simulink model "longitudinal_new"  (R2019a)
settings: Solver=VariableStepAuto  StartTime=0.0  StopTime=2000  RelTol=1e-3
values from neighbouring files (symbols this model uses):
  A = [-0.0804 0.1665 0 -9.8100 0 ... (first row only)    [longitudinaloia.m]    (also in oia.m = [-0.1245 0.0350 0.0414 -0.9962 0; -15.2138 -2.0587 0.0032 0.; state_space2tf.m = [-0.0558 -0.9968 0.0802 0.0415;0.5980 -0.1150 -0.0318 0;-3.0)
  B = [0 32.1224 ... (first row only)    [longitudinaloia.m]    (also in oia.m = [-0.0049 0.0237 ;-4.0379 0.9613; 0   0  ; -0.0568 -1.2168; 0; state_space2tf.m = [0.0073 0; -0.4750    0.0077;  0.1530    0.1430;0         0])
  C = [1          0          0          0 0;  0          1       0          0 0 ; 0       0          1          0 0; 0  0    0        1 0; 0 0 0 0 1]    [longitudinaloia.m]    (also in oia.m; state_space2tf.m = [0     1     0     0;  0     0     0     1])
  D = [0 0 ;0 0 ; 0 0 ;0   0;0 0]    [longitudinaloia.m]    (also in oia.m; state_space2tf.m = [0 0; 0 0])
libraries: simulink x3
settings Model: Creator=admin  LastModifiedBy=admin

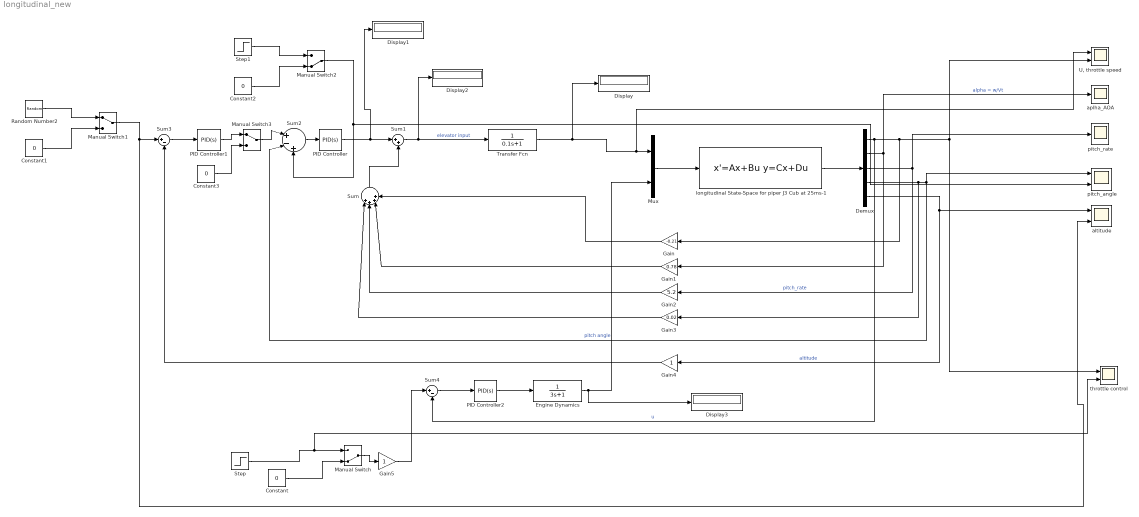
== system longitudinal_new ==
  " throttle control" : Scope  NumInputPorts=2
  Constant{,1..3} (4 alike) : Constant  Value=0
  Demux : Demux  Outputs=5
  Display{,1..3} (4 alike) : Display
  Engine Dynamics : TransferFcn  Denominator=[3 1]
  Gain : Gain  Gain=-0.21
  Gain1 : Gain  Gain=0.78
  Gain2 : Gain  Gain=5.2
  Gain3 : Gain  Gain=0.02
  Gain4 : Gain
  Gain5 : Gain
  Manual Switch : ManualSwitch  CurrentSetting=0
  Manual Switch1 : ManualSwitch
  Manual Switch2 : ManualSwitch  CurrentSetting=0
  Manual Switch3 : ManualSwitch
  Mux : Mux  Inputs=2
  PID Controller : simulink/Continuous/PID Controller  Controller=PID  Form=Parallel  TimeDomain=Continuous-time  SampleTime=-1  IntegratorMethod=Forward Euler  FilterMethod=Forward Euler  ControllerParametersSource=internal  P=0.45  I=0.4  D=0  UseFilter=on  N=100  TunerSelectOption=Transfer Function Based (PID Tuner App)  InitialConditionSource=internal  InitialConditionForIntegrator=0  InitialConditionForFilter=0  DifferentiatorICPrevScaledInput=0  ExternalReset=none  TrackingMode=off  Kt=1  LimitOutput=off  UpperSaturationLimit=inf  LowerSaturationLimit=-inf  LinearizeAsGain=on  AntiWindupMode=none  Kb=1  POutMin=[]  POutMax=[]  IOutMin=[]  IOutMax=[]  DOutMin=[]  DOutMax=[]  NOutMin=[]  NOutMax=[]  SumOutMin=[]  SumOutMax=[]  SaturationOutMin=[]  SaturationOutMax=[]  PParamMin=[]  PParamMax=[]  IParamMin=[]  IParamMax=[]  DParamMin=[]  DParamMax=[]  NParamMin=[]  NParamMax=[]  KbParamMin=[]  KbParamMax=[]  KtParamMin=[]  KtParamMax=[]  KbOutMin=[]  KbOutMax=[]  KtOutMin=[]  KtOutMax=[]  IntegratorOutMin=[]  IntegratorOutMax=[]  FilterOutMin=[]  FilterOutMax=[]  SumI1OutMin=[]  SumI1OutMax=[]  SumI2OutMin=[]  SumI2OutMax=[]  SumI3OutMin=[]  SumI3OutMax=[]  SumI4OutMin=[]  SumI4OutMax=[]  SumDOutMin=[]  SumDOutMax=[]  DifferentiatorOutMin=[]  DifferentiatorOutMax=[]  FilterDiffOutCoefMin=[]  FilterDiffOutCoefMax=[]  ReciprocalOutMin=[]  ReciprocalOutMax=[]  SumDenOutMin=[]  SumDenOutMax=[]  SumNumOutMin=[]  SumNumOutMax=[]  DivideOutMin=[]  DivideOutMax=[]  IntegratorContinuousStateAttributes=''  IntegratorStateMustResolveToSignalObject=off  IntegratorRTWStateStorageClass=Auto  FilterContinuousStateAttributes=''  FilterStateMustResolveToSignalObject=off  FilterRTWStateStorageClass=Auto  ParallelPVariant=InternalParameters  IdealPVariant=Disabled  IVariant=InternalParameters  DVariant=InternalParameters  IntegratorVariant=Continuous  SatVariant=Disabled  AWVariant=Passthrough  PCopyVariant=Disabled  TRVariant=Disabled  FdbkBlocksVariant=Forward  IdealPFdbkVariant=Disabled  SatFdbkVariant=Disabled  DerivativeFilterVariant=ContFilter  NVariant=InternalParameters  NCopyVariant=Disabled  FilterICVariant=InternalICsFilter  IntegratorICVariant=InternalICs  ExternalResetVariant=Disabled  TRSumVariant=Passthrough  SumFdbkVariant=Disabled  SumVariant=Sum_PID
  PID Controller1 : simulink/Continuous/PID Controller  Controller=PID  Form=Parallel  TimeDomain=Continuous-time  SampleTime=-1  IntegratorMethod=Forward Euler  FilterMethod=Forward Euler  ControllerParametersSource=internal  P=0.0002  I=0  D=0.02  UseFilter=on  N=100  TunerSelectOption=Transfer Function Based (PID Tuner App)  InitialConditionSource=internal  InitialConditionForIntegrator=0  InitialConditionForFilter=0  DifferentiatorICPrevScaledInput=0  ExternalReset=none  TrackingMode=off  Kt=1  LimitOutput=off  UpperSaturationLimit=inf  LowerSaturationLimit=-inf  LinearizeAsGain=on  AntiWindupMode=none  Kb=1  POutMin=[]  POutMax=[]  IOutMin=[]  IOutMax=[]  DOutMin=[]  DOutMax=[]  NOutMin=[]  NOutMax=[]  SumOutMin=[]  SumOutMax=[]  SaturationOutMin=[]  SaturationOutMax=[]  PParamMin=[]  PParamMax=[]  IParamMin=[]  IParamMax=[]  DParamMin=[]  DParamMax=[]  NParamMin=[]  NParamMax=[]  KbParamMin=[]  KbParamMax=[]  KtParamMin=[]  KtParamMax=[]  KbOutMin=[]  KbOutMax=[]  KtOutMin=[]  KtOutMax=[]  IntegratorOutMin=[]  IntegratorOutMax=[]  FilterOutMin=[]  FilterOutMax=[]  SumI1OutMin=[]  SumI1OutMax=[]  SumI2OutMin=[]  SumI2OutMax=[]  SumI3OutMin=[]  SumI3OutMax=[]  SumI4OutMin=[]  SumI4OutMax=[]  SumDOutMin=[]  SumDOutMax=[]  DifferentiatorOutMin=[]  DifferentiatorOutMax=[]  FilterDiffOutCoefMin=[]  FilterDiffOutCoefMax=[]  ReciprocalOutMin=[]  ReciprocalOutMax=[]  SumDenOutMin=[]  SumDenOutMax=[]  SumNumOutMin=[]  SumNumOutMax=[]  DivideOutMin=[]  DivideOutMax=[]  IntegratorContinuousStateAttributes=''  IntegratorStateMustResolveToSignalObject=off  IntegratorRTWStateStorageClass=Auto  FilterContinuousStateAttributes=''  FilterStateMustResolveToSignalObject=off  FilterRTWStateStorageClass=Auto  ParallelPVariant=InternalParameters  IdealPVariant=Disabled  IVariant=InternalParameters  DVariant=InternalParameters  IntegratorVariant=Continuous  SatVariant=Disabled  AWVariant=Passthrough  PCopyVariant=Disabled  TRVariant=Disabled  FdbkBlocksVariant=Forward  IdealPFdbkVariant=Disabled  SatFdbkVariant=Disabled  DerivativeFilterVariant=ContFilter  NVariant=InternalParameters  NCopyVariant=Disabled  FilterICVariant=InternalICsFilter  IntegratorICVariant=InternalICs  ExternalResetVariant=Disabled  TRSumVariant=Passthrough  SumFdbkVariant=Disabled  SumVariant=Sum_PID
  PID Controller2 : simulink/Continuous/PID Controller  Controller=PID  Form=Parallel  TimeDomain=Continuous-time  SampleTime=-1  IntegratorMethod=Forward Euler  FilterMethod=Forward Euler  ControllerParametersSource=internal  P=0.000525096772530995  I=1.12730428035271e-05  D=-0.00351336119026561  UseFilter=on  N=0.016229698913469  TunerSelectOption=Transfer Function Based (PID Tuner App)  InitialConditionSource=internal  InitialConditionForIntegrator=0  InitialConditionForFilter=0  DifferentiatorICPrevScaledInput=0  ExternalReset=none  TrackingMode=off  Kt=1  LimitOutput=off  UpperSaturationLimit=inf  LowerSaturationLimit=-inf  LinearizeAsGain=on  AntiWindupMode=none  Kb=1  POutMin=[]  POutMax=[]  IOutMin=[]  IOutMax=[]  DOutMin=[]  DOutMax=[]  NOutMin=[]  NOutMax=[]  SumOutMin=[]  SumOutMax=[]  SaturationOutMin=[]  SaturationOutMax=[]  PParamMin=[]  PParamMax=[]  IParamMin=[]  IParamMax=[]  DParamMin=[]  DParamMax=[]  NParamMin=[]  NParamMax=[]  KbParamMin=[]  KbParamMax=[]  KtParamMin=[]  KtParamMax=[]  KbOutMin=[]  KbOutMax=[]  KtOutMin=[]  KtOutMax=[]  IntegratorOutMin=[]  IntegratorOutMax=[]  FilterOutMin=[]  FilterOutMax=[]  SumI1OutMin=[]  SumI1OutMax=[]  SumI2OutMin=[]  SumI2OutMax=[]  SumI3OutMin=[]  SumI3OutMax=[]  SumI4OutMin=[]  SumI4OutMax=[]  SumDOutMin=[]  SumDOutMax=[]  DifferentiatorOutMin=[]  DifferentiatorOutMax=[]  FilterDiffOutCoefMin=[]  FilterDiffOutCoefMax=[]  ReciprocalOutMin=[]  ReciprocalOutMax=[]  SumDenOutMin=[]  SumDenOutMax=[]  SumNumOutMin=[]  SumNumOutMax=[]  DivideOutMin=[]  DivideOutMax=[]  IntegratorContinuousStateAttributes=''  IntegratorStateMustResolveToSignalObject=off  IntegratorRTWStateStorageClass=Auto  FilterContinuousStateAttributes=''  FilterStateMustResolveToSignalObject=off  FilterRTWStateStorageClass=Auto  ParallelPVariant=InternalParameters  IdealPVariant=Disabled  IVariant=InternalParameters  DVariant=InternalParameters  IntegratorVariant=Continuous  SatVariant=Disabled  AWVariant=Passthrough  PCopyVariant=Disabled  TRVariant=Disabled  FdbkBlocksVariant=Forward  IdealPFdbkVariant=Disabled  SatFdbkVariant=Disabled  DerivativeFilterVariant=ContFilter  NVariant=InternalParameters  NCopyVariant=Disabled  FilterICVariant=InternalICsFilter  IntegratorICVariant=InternalICs  ExternalResetVariant=Disabled  TRSumVariant=Passthrough  SumFdbkVariant=Disabled  SumVariant=Sum_PID
  Random Number2 : RandomNumber  SampleTime=750
  Step : Step  Time=1000  SampleTime=0
  Step1 : Step  Time=500  SampleTime=0
  Sum : Sum  Inputs=|++++
  Sum1 : Sum  Inputs=|++
  Sum2 : Sum  Inputs=|+-+
  Sum3 : Sum  Inputs=|+-
  Sum4 : Sum  Inputs=|+-
  Transfer Fcn : TransferFcn  Denominator=[0.1 1]
  "U, throttle speed" : Scope  NumInputPorts=2
  altitude : Scope  NumInputPorts=2
  aplha_AOA : Scope
  "longitudinal State-Space for piper J3 Cub at 25ms-1 " : StateSpace  A=A  B=B  C=C  D=D  InitialCondition=[0.11 0.01 0.01 0.01 0.001]
  pitch_angle : Scope  NumInputPorts=2
  pitch_rate : Scope
  wires:
  Mux/1 -> "longitudinal State-Space for piper J3 Cub at 25ms-1 "/1
  "longitudinal State-Space for piper J3 Cub at 25ms-1 "/1 -> Demux/1
  Demux/2 -> aplha_AOA/1, Gain1/1  "alpha = w/Vt"
  Demux/3 -> pitch_rate/1, Gain2/1  "pitch_rate"
  Demux/4 -> Gain3/1, Sum2/2, pitch_angle/1  "pitch angle"
  Demux/5 -> Gain4/1, altitude/1  "altitude"
  Demux/1 -> Sum4/2, Gain/1, " throttle control"/1, "U, throttle speed"/2  "u"
  Sum1/1 -> Transfer Fcn/1, Display2/1  "elevator input"
  Sum/1 -> Sum1/2
  Gain/1 -> Sum/4
  Gain1/1 -> Sum/3
  Gain2/1 -> Sum/2
  Gain3/1 -> Sum/1
  Sum2/1 -> PID Controller/1
  PID Controller/1 -> Display1/1, Sum1/1
  Transfer Fcn/1 -> Display/1, "U, throttle speed"/1, Mux/1
  Manual Switch1/1 -> Sum3/1, altitude/2
  Gain4/1 -> Sum3/2
  Engine Dynamics/1 -> Display3/1, Mux/2
  Gain5/1 -> Sum4/1
  Sum4/1 -> PID Controller2/1
  PID Controller2/1 -> Engine Dynamics/1
  Step/1 -> " throttle control"/2, Manual Switch/1
  Manual Switch/1 -> Gain5/1
  Constant/1 -> Manual Switch/2
  Random Number2/1 -> Manual Switch1/1
  Constant1/1 -> Manual Switch1/2
  Constant2/1 -> Manual Switch2/2
  Step1/1 -> Manual Switch2/1
  Sum3/1 -> PID Controller1/1
  Manual Switch2/1 -> pitch_angle/2, Sum2/3
  PID Controller1/1 -> Manual Switch3/1
  Manual Switch3/1 -> Sum2/1
  Constant3/1 -> Manual Switch3/2
